simulink model "ford"  (R2020a)
settings: Solver=VariableStepAuto  StartTime=0.0  StopTime=100.0  MaxStep=2.0  RelTol=1e-3
model workspace (MAT data in the model file):
  b = 350
  k1 = 50000
  k2 = 50000
values from neighbouring files (symbols this model uses):
  m1 = 2500    [TRUCK.mat]    (also in truck.m)
  m2 = 320    [TRUCK.mat]    (also in truck.m)
settings Model: Creator=Admin  LastModifiedBy=Admin

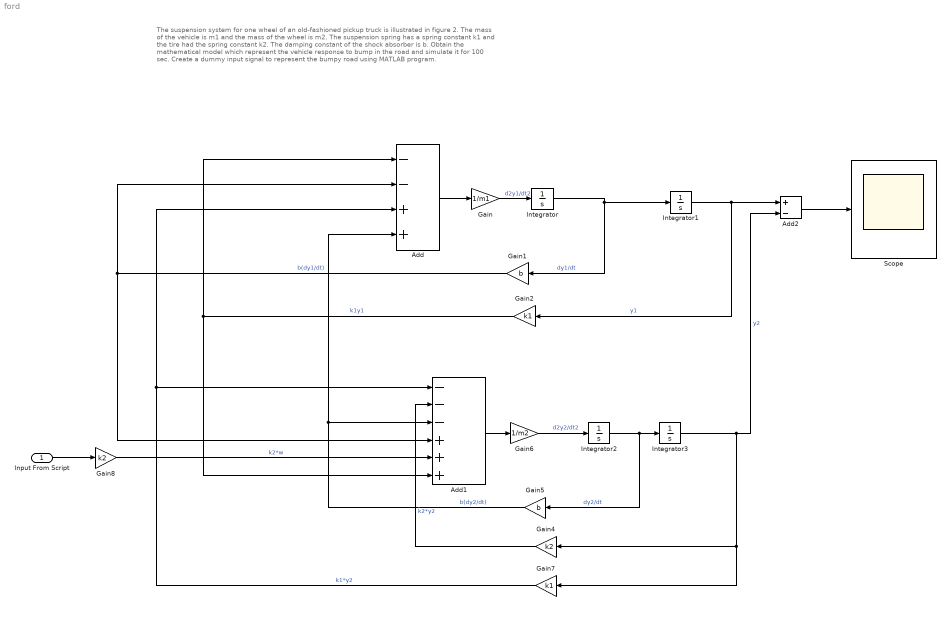
== system ford ==
  note: The suspension system for one wheel of an old-fashioned pickup truck is illustrated in figure 2. The mass of the vehicle is m1 and the mass of the wheel is m2. The suspension spring has a spring constant k1 and the tire had the spring constant k2. The damping constant of the shock absorber is b. Obtain the mathematical model which represent the vehicle response to bump in the road and simulate it for 100 sec. Create a dummy input signal to represent the bumpy road using MATLAB program.
  Input From Script : Inport
  Add : Sum  Inputs=--++
  Add1 : Sum  Inputs=---+++
  Add2 : Sum  Inputs=+-
  Gain : Gain  Gain=1/m1
  Gain1 : Gain  Gain=b
  Gain2 : Gain  Gain=k1
  Gain4 : Gain  Gain=k2
  Gain5 : Gain  Gain=b
  Gain6 : Gain  Gain=1/m2
  Gain7 : Gain  Gain=k1
  Gain8 : Gain  Gain=k2
  Integrator{,1..3} (4 alike) : Integrator
  Scope : Scope
  wires:
  Add2/1 -> Scope/1
  Gain/1 -> Integrator/1  "d2y1/dt2"
  Integrator1/1 -> Add2/1, Gain2/1  "y1"
  Input From Script/1 -> Gain8/1
  Add/1 -> Gain/1
  Gain8/1 -> Add1/5  "k2*w"
  Gain2/1 -> Add/1, Add1/6  "k1y1"
  Gain7/1 -> Add/3, Add1/1  "k1*y2"
  Gain5/1 -> Add/4, Add1/3  "b(dy2/dt)"
  Add1/1 -> Gain6/1
  Integrator2/1 -> Gain5/1, Integrator3/1  "dy2/dt"
  Gain4/1 -> Add1/2  "k2*y2"
  Gain1/1 -> Add/2, Add1/4  "b(dy1/dt)"
  Integrator3/1 -> Gain7/1, Gain4/1, Add2/2  "y2"
  Gain6/1 -> Integrator2/1  "d2y2/dt2"
  Integrator/1 -> Integrator1/1, Gain1/1  "dy1/dt"
